simulink model "model_davide"  (R2022b)
settings: Solver=VariableStepAuto  StartTime=0.0  StopTime=40  RelTol=1e-3
undefined symbols (not defined in the file): Aw, I, Ir, Kd, Ki, Kp, m, pos_ref, psi, t_ref, vel_ref
libraries: vrlib x4, slpidlib x4
settings Model: Creator=iris  LastModifiedBy=d066566
settings SolverCC: AlgebraicLoopSolver=TrustRegion
settings DebuggingCC: UnconnectedInputMsg=warning  UnconnectedOutputMsg=warning  UnconnectedLineMsg=warning
settings ModelReferenceCC: EnableRefExpFcnMdlSchedulingChecks=on
settings RTWCC: DLArmComputeVersion=19.05

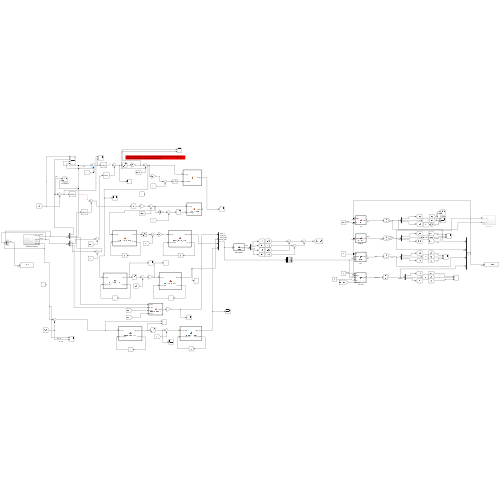
[thumbnail: Simulink's stored preview of the top-level diagram]
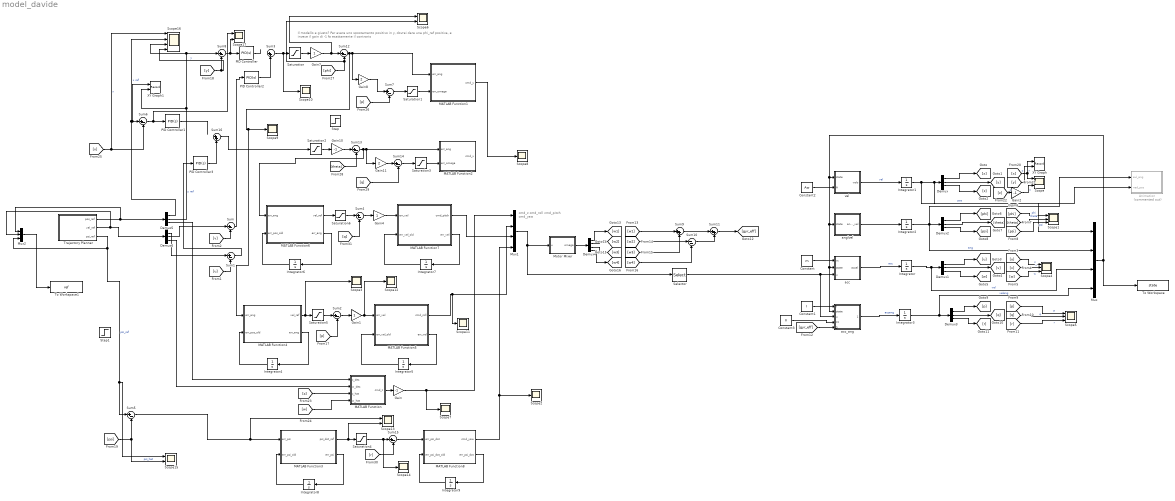
== system model_davide ==
  note: cmd_z
      | cmd_roll
      | cmd_pitch
      | cmd_yaw
  note: Il modello e giusto? Per avere uno spostamento positivo in y, dovrei dare una phi_ref positiva, e invece il gain di -1 fa esattamente il contrario
  Animation : Subsystem  Commented=on
  Constant : Constant  Value=m
  Constant1 : Constant  Value=I
  Constant2 : Constant  Value=Aw
  Constant3 : Constant  Value=Ir
  Demux{,1..3,5..6} (6 alike) : Demux  Outputs=3
  Demux4 : Demux
  Gain : Gain  Gain=-1
  Gain1 : Gain
  Gain10 : Gain  Gain=-1
  Gain11 : Gain  Gain=2
  Gain2 : Gain  Gain=-1
  Gain4 : Gain
  Gain7 : Gain
  Gain8 : Gain  Gain=2
  Integrator{,1..3} (4 alike) : Integrator  InitialCondition=[0,0,0]
  Integrator{4..9} (6 alike) : Integrator
  MATLAB Function : MATLAB Function  TreatAsAtomicUnit=on
  MATLAB Function1 : MATLAB Function  TreatAsAtomicUnit=on
  MATLAB Function2 : MATLAB Function  TreatAsAtomicUnit=on
  MATLAB Function3 : MATLAB Function  TreatAsAtomicUnit=on
  MATLAB Function4 : MATLAB Function  TreatAsAtomicUnit=on
  MATLAB Function5 : MATLAB Function  TreatAsAtomicUnit=on
  MATLAB Function6 : MATLAB Function  TreatAsAtomicUnit=on
  MATLAB Function7 : MATLAB Function  TreatAsAtomicUnit=on
  MATLAB Function8 : MATLAB Function  TreatAsAtomicUnit=on
  Motor Mixer : MATLAB Function  TreatAsAtomicUnit=on
  Mux : Mux
  Mux1 : Mux
  Mux2 : Mux  Inputs=3
  PID Controller{,1..3} (4 alike) : slpidlib/PID Controller  Controller=PID  Form=Parallel  TimeDomain=Continuous-time  UseExternalTs=off  SampleTime=-1  IntegratorMethod=Forward Euler  FilterMethod=Forward Euler  ControllerParametersSource=internal  P=Kp  I=Ki  UseKiTs=off  D=Kd  N=100  UseFilter=on  TunerSelectOption=Transfer Function Based (PID Tuner App)  InitialConditionSource=internal  InitialConditionForIntegrator=0  InitialConditionForFilter=0  DifferentiatorICPrevScaledInput=0  ExternalReset=none  TrackingMode=off  Kt=1  LimitOutput=off  SatLimitsSource=internal  UpperSaturationLimit=inf  LowerSaturationLimit=-inf  LinearizeAsGain=on  AntiWindupMode=none  Kb=1  LimitIntegrator=off  UpperIntegratorSaturationLimit=inf  LowerIntegratorSaturationLimit=-inf  POutMin=[]  POutMax=[]  IOutMin=[]  IOutMax=[]  DOutMin=[]  DOutMax=[]  NOutMin=[]  NOutMax=[]  SumOutMin=[]  SumOutMax=[]  SaturationOutMin=[]  SaturationOutMax=[]  PParamMin=[]  PParamMax=[]  IParamMin=[]  IParamMax=[]  DParamMin=[]  DParamMax=[]  NParamMin=[]  NParamMax=[]  KbParamMin=[]  KbParamMax=[]  KtParamMin=[]  KtParamMax=[]  KbOutMin=[]  KbOutMax=[]  KtOutMin=[]  KtOutMax=[]  IntegratorOutMin=[]  IntegratorOutMax=[]  FilterOutMin=[]  FilterOutMax=[]  SumI1OutMin=[]  SumI1OutMax=[]  SumI2OutMin=[]  SumI2OutMax=[]  SumI3OutMin=[]  SumI3OutMax=[]  SumI4OutMin=[]  SumI4OutMax=[]  SumDOutMin=[]  SumDOutMax=[]  DifferentiatorOutMin=[]  DifferentiatorOutMax=[]  FilterDiffOutCoefMin=[]  FilterDiffOutCoefMax=[]  ReciprocalOutMin=[]  ReciprocalOutMax=[]  SumDenOutMin=[]  SumDenOutMax=[]  SumNumOutMin=[]  SumNumOutMax=[]  DivideOutMin=[]  DivideOutMax=[]  UdiffTsProdOutMin=[]  UdiffTsProdOutMax=[]  NTsProdOutMin=[]  NTsProdOutMax=[]  UintegralTsProdOutMin=[]  UintegralTsProdOutMax=[]  UngainTsProdOutMin=[]  UngainTsProdOutMax=[]  ClampingZeroOutDataTypeStr=Inherit: Inherit via back propagation  ClampingZeroOutMin=[]  ClampingZeroOutMax=[]  FilterDenConstantOutDataTypeStr=Inherit: Inherit via back propagation  FilterDenConstantOutMin=[]  FilterDenConstantOutMax=[]  PCopyOutDataTypeStr=Inherit: Inherit via back propagation  PCopyOutMin=[]  PCopyOutMax=[]  NCopyOutDataTypeStr=Inherit: Inherit via back propagation  NCopyOutMin=[]  NCopyOutMax=[]  IntegratorContinuousStateAttributes=''  IntegratorStateMustResolveToSignalObject=off  IntegratorRTWStateStorageClass=Auto  FilterContinuousStateAttributes=''  FilterStateMustResolveToSignalObject=off  FilterRTWStateStorageClass=Auto  ParallelPVariant=InternalParameters  IdealPVariant=Disabled  IVariant=InternalParameters  DVariant=InternalParameters  IntegratorVariant=Continuous  SatVariant=Disabled  AWVariant=Passthrough  PCopyVariant=Disabled  TRVariant=Disabled  FdbkBlocksVariant=Forward  IdealPFdbkVariant=Disabled  SatFdbkVariant=Disabled  DerivativeFilterVariant=ContFilter  NVariant=InternalParameters  NCopyVariant=Disabled  FilterICVariant=InternalICsFilter  IntegratorICVariant=InternalICs  ExternalResetVariant=Disabled  TRSumVariant=Passthrough  SumFdbkVariant=Disabled  SumVariant=Sum_PID  TsampFilterVariant=InternalTs  TsampNgainVariant=Passthrough  TsampIntegralVariant=Passthrough  ExternalSaturationOutDataTypeStr=Inherit: Same as second input
  Saturation : Saturate  UpperLimit=pi/6  LowerLimit=-pi/6
  Saturation1 : Saturate
  Saturation2 : Saturate  UpperLimit=pi/8  LowerLimit=-pi/8
  Saturation3 : Saturate
  Saturation4 : Saturate  UpperLimit=2 / 3* pi  LowerLimit=-2 / 3 *pi
  Saturation5 : Saturate  UpperLimit=3  LowerLimit=-3
  Saturation6 : Saturate  UpperLimit=3  LowerLimit=-3
  Scope{,1,4..5} (4 alike) : Scope  NumInputPorts=3
  Scope{2..3,7..12,14} (9 alike) : Scope
  Scope{6,13,15,17} (4 alike) : Scope  NumInputPorts=2
  Scope16 : Scope  NumInputPorts=4
  Selector : Selector  InputPortWidth=4  IndexOptions=Index vector (dialog)  Indices=[1 2 3 4]  OutputSizes=1
  Step : Step  Time=5  After=-pi/8  SampleTime=0
  Step1 : Step  Time=2  After=pi  SampleTime=0
  Sum{,1..2,4..8,12..15} (12 alike) : Sum  Inputs=|+-
  Sum10 : Sum  Inputs=|--
  Sum{3,9,11,16} (4 alike) : Sum  Inputs=|++
  To Workspace : ToWorkspace  VariableName=state  SampleTime=-1
  To Workspace1 : ToWorkspace  VariableName=ref  SampleTime=-1
  Trajectory Planner : Subsystem
  XY Graph : Record  FileSettingsInternal="{\"entries\":[{\"content\":{\"excelSettings\":{\"content\":{},\"type\":\"Streamout.ExcelSettings\"}},\"type\":\"Streamout.FileSettingStorage\",\"uuid\":\"8b606f2d-9703-420a-beb1-d133885c238d\"}],\"packageUris\":[\"http://schema.mathworks.com/mf0/streamout_blocks/R2020a\"],\"version\":\"1.0\"}"  Layout=[1 1]  SignalsInternal="{\"entries\":[{\"content\":{\"signals\":[{\"content\":{\"blockPath\":[\"model_davide/XY Graph\"],\"channel\":[],\"dimensions\":[1],\"domain\":\"model_davide/XY Graph\",\"lineColor\":\"#a2142f\",\"plots\":[1],\"port\":1,\"sid\":[\"\"],\"signalID\":2972,\"signalName\":\"x\"},\"type\":\"RecordBlkView.Signal\",\"uuid\":\"0564af82-42f0-40b4-a488-d10341f20b41\"},{\"content\":{\"blockPath\":[\"model_davide/XY Graph\"],\"channel\":[],\"dimensions\":[1],\"domain\":\"model_davide/XY Graph\",\"lineColor\":\"#139fff\",\"plots\":[1],\"port\":2,\"sid\":[\"\"],\"signalID\":2976,\"signalName\":\"y\"},\"type\":\"RecordBlkView.Signal\",\"uuid\":\"9ac8722f-5668-4699-b1ca-3924ff1782ea\"}]},\"type\":\"RecordBlkView.InputSignals\",\"uuid\":\"f3bc4df6-649b-4f3a-a8dc-c16e176b0357\"}],\"packageUris\":[\"http://schema.mathworks.com/mf0/streamout_blocks/R2020a\"],\"version\":\"1.0\"}"  VisualizationBindings="{\"xyplotplugin\":{\"info\":[{\"series\":[{\"bindingParametersList\":[{\"parameter\":\"X-Axis\",\"signalID\":2972,\"signalName\":\"x\"},{\"parameter\":\"Y-Axis\",\"signalID\":2976,\"signalName\":\"y\"}],\"seriesID\":63110}],\"subplotID\":1}]}}"  CompatibilityTag=XY  st=-1
  XY Graph1 : Record  FileSettingsInternal="{\"entries\":[{\"content\":{\"excelSettings\":{\"content\":{},\"type\":\"Streamout.ExcelSettings\"}},\"type\":\"Streamout.FileSettingStorage\",\"uuid\":\"0285df6e-5a15-4ea3-a0ef-6602bf7d78b3\"}],\"packageUris\":[\"http://schema.mathworks.com/mf0/streamout_blocks/R2020a\"],\"version\":\"1.0\"}"  Layout=[1 1]  SignalsInternal="{\"entries\":[{\"content\":{\"signals\":[{\"content\":{\"blockPath\":[\"model_davide/XY Graph1\"],\"channel\":[],\"dimensions\":[1,1],\"domain\":\"model_davide/XY Graph1\",\"lineColor\":\"#a2142f\",\"plots\":[1],\"port\":1,\"sid\":[\"\"],\"signalID\":2980,\"signalName\":\"x ref\"},\"type\":\"RecordBlkView.Signal\",\"uuid\":\"36f7bd12-7292-478b-980e-bc441240de97\"},{\"content\":{\"blockPath\":[\"model_davide/XY Graph1\"],\"channel\":[],\"dimensions\":[1,1],\"domain\":\"model_davide/XY Graph1\",\"lineColor\":\"#139fff\",\"plots\":[1],\"port\":2,\"sid\":[\"\"],\"signalID\":2984,\"signalName\":\"y ref\"},\"type\":\"RecordBlkView.Signal\",\"uuid\":\"4182ead5-5d37-44fc-8076-4a3e7f86adc1\"}]},\"type\":\"RecordBlkView.InputSignals\",\"uuid\":\"355609ca-6548-483a-8627-9d9e152220d5\"}],\"packageUris\":[\"http://schema.mathworks.com/mf0/streamout_blocks/R2020a\"],\"version\":\"1.0\"}"  VisualizationBindings="{\"xyplotplugin\":{\"info\":[{\"series\":[{\"bindingParametersList\":[{\"parameter\":\"X-Axis\",\"signalID\":2980,\"signalName\":\"x ref\"},{\"parameter\":\"Y-Axis\",\"signalID\":2984,\"signalName\":\"y ref\"}],\"seriesID\":17628}],\"subplotID\":1}]}}"  CompatibilityTag=XY  st=-1
  acc : MATLAB Function  TreatAsAtomicUnit=on
  acc_ang : MATLAB Function  TreatAsAtomicUnit=on
  anglvel : MATLAB Function  TreatAsAtomicUnit=on
  vel : MATLAB Function  TreatAsAtomicUnit=on
  wires:
  Constant/1 -> acc/1(m)
  Constant1/1 -> acc_ang/1(I)
  Motor Mixer/1(omega) -> Demux4/1
  Demux4/1 -> [w1]
  Demux4/2 -> [w2]
  Demux4/3 -> [w3]
  Demux4/4 -> [w4]
  [v] -> Sum/2
  [u] -> Sum1/2
  Sum5/1 -> Scope13/1, MATLAB Function3/1("err_psi ")
  [psi] -> Sum5/2, Scope15/2  "psi_hat"
  MATLAB Function/1(cmd_z) -> Gain/1
  Mux1/1 -> Selector/1, Motor Mixer/1(u)
  Integrator3/1 -> Mux/4, Demux3/1  "velang"
  Demux/3 -> [z]
  Integrator/1 -> Mux/3, Demux1/1  "vel"
  Demux3/3 -> [r]
  Integrator2/1 -> Animation/1(eul_ang), Demux2/1, Mux/2  "ang"
  acc_ang/1(accel_ang) -> Integrator3/1  "accang"
  Demux/1 -> [x]
  Demux2/1 -> [phi]
  Demux2/3 -> [psi]
  Demux1/3 -> [w]
  Demux3/1 -> [p]
  anglvel/1(angular_vel) -> Integrator2/1
  Integrator1/1 -> Animation/2(ned_pos), Mux/1, Demux/1  "pos"
  Demux1/1 -> [u]
  Demux3/2 -> [q]
  Demux/2 -> [y]
  Demux1/2 -> [v]
  Demux2/2 -> [theta]
  acc/1(accel) -> Integrator/1  "acc"
  vel/1(velo) -> Integrator1/1  "vel"
  Mux/1 -> acc_ang/2(state), acc/2(state), anglvel/1(state), vel/1(state), To Workspace/1
  [x] -> XY Graph/1, Scope/1  "x"
  [y] -> Scope/2, XY Graph/2  "y"
  [z] -> Gain2/1  "z"
  Selector/1 -> acc/3(u), acc_ang/3(u)
  Gain/1 -> Mux1/1, Scope7/1
  Gain2/1 -> Scope/3  "z"
  [phi] -> Scope1/1  "phi"
  [theta] -> Scope1/2  "theta"
  [psi] -> Scope1/3  "psi"
  Trajectory Planner/1(pos_ref) -> Mux2/1, Demux5/1
  Demux5/3 -> MATLAB Function/1(z_des)
  Trajectory Planner/2(vel_ref) -> Mux2/2, Demux6/1
  Demux6/1 -> Sum1/1
  Demux6/2 -> Sum/1
  Demux6/3 -> MATLAB Function/2(w_des)
  [w1] -> Sum9/1
  [w3] -> Sum9/2
  [w2] -> Sum10/1
  [w4] -> Sum10/2
  Sum10/1 -> Sum11/2
  Sum9/1 -> Sum11/1
  Sum11/1 -> [gyr_eff]
  [gyr_eff] -> acc_ang/5(gyr_eff)
  Constant2/1 -> vel/2(A)
  Constant3/1 -> acc_ang/4(Irz)
  [u] -> Scope4/1  "u"
  [v] -> Scope4/2  "v"
  [w] -> Scope4/3  "w"
  [p] -> Scope5/1  "p"
  [q] -> Scope5/2  "q"
  [r] -> Scope5/3  "r"
  [z] -> MATLAB Function/3(z_hat)
  [w] -> MATLAB Function/4(w_hat)
  [x] -> Scope16/1, Sum6/2  "x"
  Sum6/1 -> Scope17/1, PID Controller1/1
  MATLAB Function1/1(cmd_y) -> Scope8/1
  [phi] -> Scope6/2, Sum12/2
  Saturation1/1 -> MATLAB Function1/2(err_omega)
  Sum12/1 -> MATLAB Function1/1(err_ang), Gain8/1, Scope9/1, MATLAB Function4/1("err_ang ")
  Gain8/1 -> Sum7/1
  Gain7/1 -> Scope6/1, Sum12/1
  [p] -> Sum7/2
  Saturation/1 -> Gain7/1
  Sum7/1 -> Saturation1/1
  PID Controller1/1 -> ?
  Saturation2/1 -> Gain10/1
  [theta] -> Sum13/2
  Gain11/1 -> Sum14/1
  Sum14/1 -> Saturation3/1
  Saturation3/1 -> MATLAB Function2/2(err_omega)
  [q] -> Sum14/2
  Gain10/1 -> Sum13/1
  [r] -> Sum15/2
  MATLAB Function3/1(psi_dot_ref) -> Scope13/2, Saturation4/1
  MATLAB Function4/2(err_ang) -> Integrator4/1
  Integrator4/1 -> MATLAB Function4/2(err_pos_old)
  MATLAB Function5/2(err_vel) -> Integrator5/1
  Integrator5/1 -> MATLAB Function5/2(err_vel_old)
  MATLAB Function4/1(vel_ref) -> Scope3/1, Saturation5/1
  Sum2/1 -> Gain1/1
  [p] -> Sum2/2
  Saturation5/1 -> Sum2/1
  Gain1/1 -> Scope12/1, MATLAB Function5/1("err_vel ")
  Demux5/1 -> Scope16/2, XY Graph1/1, Sum6/1  "x ref"
  Demux5/2 -> XY Graph1/2, Sum8/1, Scope16/3  "y ref"
  MATLAB Function5/1(cmd_roll) -> Mux1/2, Scope11/1
  Sum8/1 -> Scope17/2, PID Controller/1
  Sum3/1 -> Scope10/1, Saturation/1
  PID Controller/1 -> ?
  Sum/1 -> PID Controller2/1
  PID Controller2/1 -> Sum3/2
  Sum13/1 -> MATLAB Function6/1("err_ang "), Gain11/1, MATLAB Function2/1(err_ang)
  MATLAB Function6/1(vel_ref) -> Saturation6/1
  Gain4/1 -> MATLAB Function7/1("err_vel ")
  Integrator6/1 -> MATLAB Function6/2(err_pos_old)
  [q] -> Sum4/2
  MATLAB Function7/2(err_vel) -> Integrator7/1
  Saturation6/1 -> Sum4/1
  Sum4/1 -> Gain4/1
  MATLAB Function6/2(err_ang) -> Integrator6/1
  Integrator7/1 -> MATLAB Function7/2(err_vel_old)
  Sum16/1 -> Saturation2/1
  PID Controller3/1 -> Sum16/2
  Sum1/1 -> PID Controller3/1
  MATLAB Function7/1(cmd_pitch) -> Mux1/3
  MATLAB Function3/2(err_psi) -> Integrator8/1
  Integrator8/1 -> MATLAB Function3/2(err_psi_old)
  Saturation4/1 -> Scope14/1, Sum15/1
  Sum15/1 -> MATLAB Function8/1("err_psi_dot ")
  MATLAB Function8/1(cmd_yaw) -> Scope2/1, Mux1/4
  MATLAB Function8/2(err_psi_dot) -> Integrator9/1
  Integrator9/1 -> MATLAB Function8/2(err_psi_dot_old)
  Trajectory Planner/3(psi_ref) -> Scope15/1, Sum5/1, Mux2/3  "psi_ref"
  [y] -> Scope16/4, Sum8/2  "y"
  Mux2/1 -> To Workspace1/1

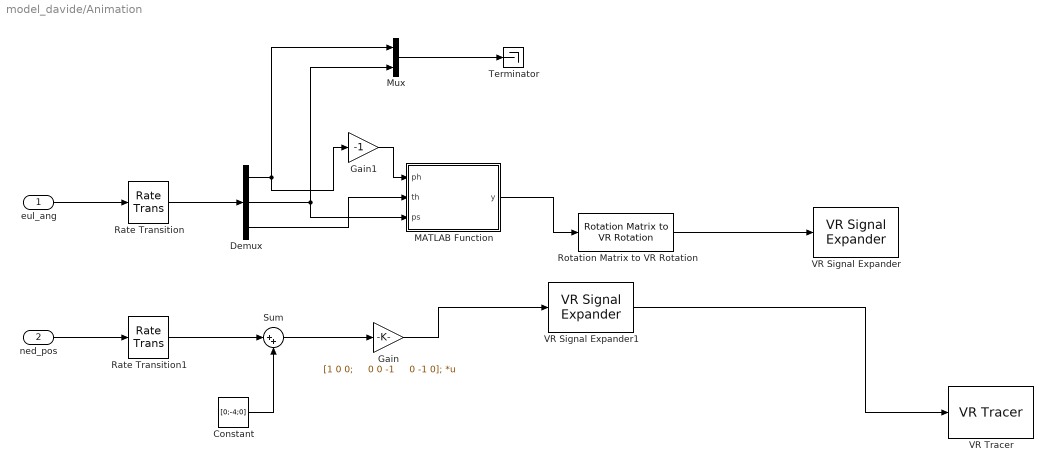
== system model_davide/Animation ==
  eul_ang : Inport
  ned_pos : Inport  Port=2
  Constant : Constant  Value=[0;-4;0]
  Demux : Demux  Outputs=3
  Gain : Gain  Gain=|  Multiplication=Matrix(K*u)
      | [1 0 0;
      |     0 0 -1
      |     0 -1 0];
  Gain1 : Gain  Gain=-1
  MATLAB Function : MATLAB Function  TreatAsAtomicUnit=on
  Mux : Mux  Inputs=2
  Rate Transition : RateTransition  OutPortSampleTime=0.1
  Rate Transition1 : RateTransition  OutPortSampleTime=0.1
  Rotation Matrix to VR Rotation : vrlib/Utilities/Rotation Matrix to VR Rotation  maxzero=1e-12
  Sum : Sum  Inputs=|++
  Terminator : Terminator
  VR Signal Expander : vrlib/VR Signal Expander  outwidth=4  outidx=[1:4]
  VR Signal Expander1 : vrlib/VR Signal Expander  outwidth=3  outidx=[1:3]
  VR Tracer : vrlib/VR Tracer  VrmlFile=uav_scene.x3dv  MarkerName=Sphere  UseLines=on  UseTriads=on  MarkerScale=[0.1 0.1 0.1]  MarkerColorSelection=Selected from color list  MarkerColor=red  rgbval=[1 0 0]  Ts=0.5  ForceViewerOpen=off  ConnectPlane=off  PlaneCoeff=[0 1 0 0]  ConnectPoint=None  PointCoord=[0 0 0]
  wires:
  ned_pos/1 -> Rate Transition1/1
  eul_ang/1 -> Rate Transition/1
  Demux/1 -> Gain1/1, Mux/1
  Rotation Matrix to VR Rotation/1 -> VR Signal Expander/1
  Rate Transition1/1 -> Sum/1
  Rate Transition/1 -> Demux/1
  Mux/1 -> Terminator/1
  VR Signal Expander1/1 -> VR Tracer/1
  Gain/1 -> VR Signal Expander1/1
  MATLAB Function/1(y) -> Rotation Matrix to VR Rotation/1
  Demux/3 -> MATLAB Function/2(th)
  Demux/2 -> MATLAB Function/3(ps), Mux/2
  Gain1/1 -> MATLAB Function/1(ph)
  Sum/1 -> Gain/1
  Constant/1 -> Sum/2

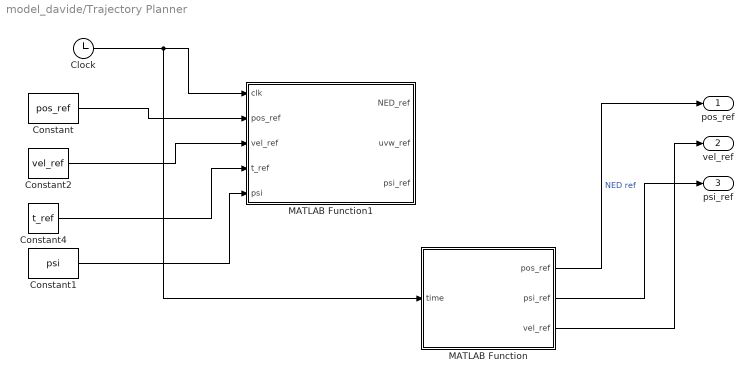
== system model_davide/Trajectory Planner ==
  Clock : Clock
  Constant : Constant  Value=pos_ref
  Constant1 : Constant  Value=psi
  Constant2 : Constant  Value=vel_ref
  Constant4 : Constant  Value=t_ref
  MATLAB Function : MATLAB Function  TreatAsAtomicUnit=on
  MATLAB Function1 : MATLAB Function  TreatAsAtomicUnit=on
  pos_ref : Outport
  vel_ref : Outport  Port=2
  psi_ref : Outport  Port=3
  wires:
  Constant/1 -> MATLAB Function1/2(pos_ref)
  Constant2/1 -> MATLAB Function1/3(vel_ref)
  Constant4/1 -> MATLAB Function1/4(t_ref)
  Clock/1 -> MATLAB Function/1(time), MATLAB Function1/1(clk)
  Constant1/1 -> MATLAB Function1/5(psi)
  MATLAB Function/1(pos_ref) -> pos_ref/1  "NED ref"
  MATLAB Function/3(vel_ref) -> vel_ref/1
  MATLAB Function/2(psi_ref) -> psi_ref/1

== matlab function model_davide/MATLAB Function3 ==
  data: err_psi input; psi_dot_ref output; err_psi_old input; err_psi output
function [ psi_dot_ref, err_psi ] = yaw_control_outer(err_psi, err_psi_old)
    
    lambda_outer = 3;%0.5;%0.07;
    K_outer = 1;%2;%0.8;
    sigma_outer = err_psi + lambda_outer * err_psi_old;
    psi_dot_ref = K_outer * tanh(sigma_outer);
end

== matlab function model_davide/MATLAB Function4 ==
  data: err_ang input; vel_ref output; err_pos_old input; err_ang output
function [ vel_ref, err_ang ] = roll_control_outer(err_ang, err_pos_old)

    lambda_outer = 7; %0.1
    K_outer = 4;%20
    sigma_outer = err_ang + lambda_outer * err_pos_old;
    vel_ref = K_outer * tanh(sigma_outer);
    
end

== matlab function model_davide/MATLAB Function5 ==
  data: err_vel input; cmd_roll output; err_vel_old input; err_vel output
function [ cmd_roll, err_vel ] = roll_control_inner(err_vel, err_vel_old)

    lambda_inner = 10; % 0.2
    K_inner = 13; % 5 
    sigma_inner = err_vel + lambda_inner * err_vel_old;
    cmd_roll = K_inner * tanh(sigma_inner);
end

== matlab function model_davide/MATLAB Function6 ==
  data: err_ang input; vel_ref output; err_pos_old input; err_ang output
function [ vel_ref, err_ang ] = pitch_control_outer(err_ang, err_pos_old)

    lambda_outer = 1;%0.1;
    K_outer = 4;%20;
    sigma_outer = err_ang + lambda_outer * err_pos_old;
    vel_ref = K_outer * tanh(sigma_outer);
    
end

== matlab function model_davide/MATLAB Function7 ==
  data: err_vel input; cmd_pitch output; err_vel_old input; err_vel output
function [ cmd_pitch, err_vel ] = pitch_control_inner(err_vel, err_vel_old)

    lambda_inner = 11;%0.2;
    K_inner = 13;%5;
    sigma_inner = err_vel + lambda_inner * err_vel_old;
    cmd_pitch = K_inner * tanh(sigma_inner);
end

== matlab function model_davide/MATLAB Function8 ==
  data: err_psi_dot input; cmd_yaw output; err_psi_dot_old input; err_psi_dot output
function [ cmd_yaw, err_psi_dot ] = roll_control_inner(err_psi_dot, err_psi_dot_old)

    lambda_inner = 7;%0.1;
    K_inner = 10;%2;
    sigma_inner = err_psi_dot + lambda_inner * err_psi_dot_old;
    cmd_yaw = K_inner * tanh(sigma_inner);
end

== matlab function model_davide/vel ==
  data: state input; velo output; A input
function velo = vel(state, A)

ph = state(4);
th = state(5);
ps = state(6);

Rot_mat = [cos(th)*cos(ps) sin(ph)*sin(th)*cos(ps)-cos(ph)*sin(ps) cos(ph)*sin(th)*cos(ps)+sin(ph)*sin(ps);
    cos(th)*sin(ps) sin(ph)*sin(th)*sin(ps)+cos(ph)*cos(ps) cos(ph)*sin(th)*sin(ps)-sin(ph)*cos(ps);
    -sin(th) sin(ph)*cos(th) cos(ph)*cos(th)]; % body to NED

velo = Rot_mat*state(7:9);
% xdot = velo(1);
% ydot = velo(2);
% zdot = velo(3);

== matlab function model_davide/Trajectory Planner/MATLAB Function ==
  data: time input; pos_ref output; psi_ref output; vel_ref output
function [ pos_ref, psi_ref,vel_ref ] = fcn(time)

%     pos_ref = 0.5 * [ sin(2 * pi * time / 15) - 1, cos(2 * pi * time / 15), 0.1 * time ];
%     psi_ref = -0.1 * time;
    psi_ref = time * 2 * pi / 15;
    pos_ref = [ 1*cos(time * 2 * pi / 15 - pi/2)', 1*sin(time * 2 * pi / 15 - pi/2)' + 1, -0.1 * time ];
    vel_ref = [ 2 * pi / 15, 0 , -0.1 ];
%     psi_ref = time *0.1;
%     pos_ref = [ 10*cos(time * 0.1)' + 10, 10*sin(time * 0.1)' + 10, -0.1 * time ];

end

== matlab function model_davide/acc ==
  data: m input; state input; u input; accel output
function accel = acc(m,state,u)


ph = state(4);
th = state(5);
ps = state(6);
udot = -1/m*(cos(ph)*sin(th)*cos(ps)+sin(ph)*sin(ps))*u(1);
vdot = -1/m*(cos(ph)*sin(th)*sin(ps)-sin(ph)*cos(ps))*u(1);
wdot = 9.81 - 1/m*(cos(ph)*cos(th))*u(1);

accel = [udot
         vdot
         wdot];

== matlab function model_davide/anglvel ==
  data: state input; angular_vel output
function angular_vel = angvel(state)

ph = state(4);
th = state(5);
ps = state(6);
p = state(10);
q = state(11);
r = state(12);

phi_dot = p + (sin(ph)*tan(th))*q - (cos(ph)*tan(th))*r;
theta_dot = cos(ph)*q + sin(ph)*r;
psi_dot = -1*(sin(ph)*sec(th)*q) + (cos(ph)*sec(th))*r;


% angular_vel(1) = phi_dot;
% angular_vel(2) = theta_dot;
% angular_vel(3) = psi_dot;
angular_vel = [phi_dot,theta_dot,psi_dot];

== matlab function model_davide/acc_ang ==
  data: I input; state input; u input; Irz input; accel_ang output; gyr_eff input
function accel_ang = acc_ang(I,state,u, Irz, gyr_eff)

p = state(10);
q = state(11);
r = state(12);
T = u(1);
tau_x = u(2,1);
tau_y = u(3,1);
tau_z = u(4,1);

Ix = I(1,1);
Iy = I(2,2);
Iz = I(3,3);
Ixy = I(1,2);
Ixz = I(1,3);
Iyz = I(2,3);

pdot = (Iy-Iz)/Ix*q*r + 1/Ix*tau_x - gyr_eff*Irz/Ix;
qdot = (Iz-Ix)/Iy*p*r + 1/Iy*tau_y - gyr_eff*Irz/Iy;
rdot = (Ix-Iy)/Iz*p*q + 1/Iz*tau_z;


accel_ang = [pdot
             qdot
             rdot];

== matlab function model_davide/Motor Mixer ==
  data: u input; omega output
function omega = mixer(u)

k = 1;
l = 0.25;
b = 1;

mat = [k k k k;
      0 l*k 0 -l*k;
      l*k 0 -l*k 0;
      b -b b -b];
  
om = u\mat;
omega = sqrt(abs(om));

== matlab function model_davide/MATLAB Function ==
  data: z_des input; cmd_z output; w_des input; z_hat input; w_hat input
function cmd_z = altitude_control(z_des, w_des, z_hat, w_hat)

    lambda = 10;
    K = 40;
    sigma = w_hat - w_des + lambda*(z_hat - z_des);
    cmd_z = -K * tanh(sigma);
end

== matlab function model_davide/Animation/MATLAB Function ==
  data: ph input; y output; th input; ps input
function y = fcn(ph,th,ps)

Rb_ned = [ cos(th)*cos(ps), cos(th)*sin(ps), -sin(th)
            -cos(ph)*sin(ps) + sin(ph)*sin(th)*cos(ps), cos(ph)...
                *cos(ps) + sin(ph)*sin(th)*sin(ps), sin(ph)*cos(th)
            sin(ph)*sin(ps) + cos(ph)*sin(th)*cos(ps), -sin(ph)...
            *cos(ps) + cos(ph)*sin(th)*sin(ps), cos(ph)*cos(th) ];
Rx = [1 0 0;
    0 1 0
    0 0 1];
        
y = Rx*Rb_ned';

== matlab function model_davide/Trajectory Planner/MATLAB Function1 ==
  data: clk input; NED_ref output; pos_ref input; vel_ref input; t_ref input; uvw_ref output; psi_ref output; psi input
function [ NED_ref, uvw_ref, psi_ref]  = trajectoryPlanner(clk,pos_ref,vel_ref,t_ref,psi)

currTime = find(clk >= t_ref);
NED_ref = pos_ref(currTime(end),:)';
uvw_ref = vel_ref(currTime(end),:)';
psi_ref = psi(currTime(end),:)';

end

== matlab function model_davide/MATLAB Function2 ==
  data: err_ang input; cmd_x output; err_omega input
function cmd_x = pitch_control(err_ang, err_omega)
    
    sigmoid = @(in) 1 / (1 + exp(-in));
    lambda2 = 10;
    K = 2;
    sigma = err_omega + lambda2 * err_ang;
    cmd_x = -(-K * tanh(sigma));
    
end

== matlab function model_davide/MATLAB Function1 ==
  data: cmd_y output; err_ang input; err_omega input
function cmd_y = roll_control(err_ang, err_omega)
    
    sigmoid = @(in) 1 / (1 + exp(-in));
    lambda2 = 10;
    K = 2;
    sigma = err_omega + lambda2 * err_ang;
    cmd_y = -(-K * tanh(sigma));
    
end
